simulink model "untitled"  (R2025b)
settings: Solver=VariableStepAuto  StartTime=0.0  StopTime=10.0  RelTol=1e-3
settings Model: Creator=mahesh  LastModifiedBy=mahesh

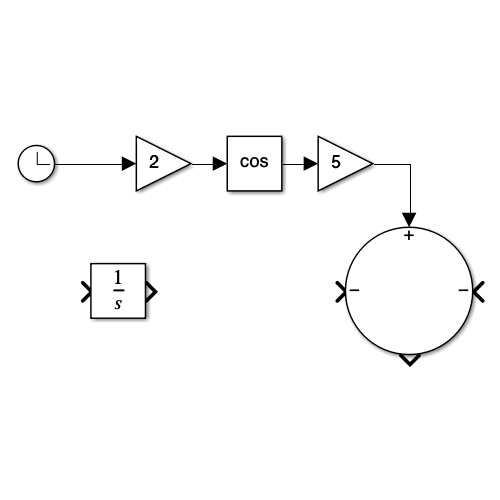
[thumbnail: Simulink's stored preview of the top-level diagram]
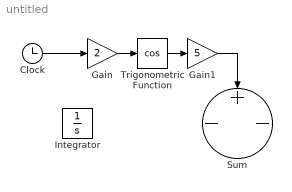
== system untitled ==
  Clock : Clock
  Gain : Gain  Gain=2
  Gain1 : Gain  Gain=5
  Integrator : Integrator
  Sum : Sum  Inputs=-+-
  Trigonometric Function : Trigonometry  Operator=cos
  wires:
  Gain/1 -> Trigonometric Function/1
  Clock/1 -> Gain/1
  Trigonometric Function/1 -> Gain1/1
  Gain1/1 -> Sum/2
